simulink model "multiplex"  (R2020a)
settings: Solver=ode45  StartTime=0.0  StopTime=tiemposimu  RelTol=1e-3  EnableMultiTasking=on
values from neighbouring files (symbols this model uses):
  Atenuacion_canal = 22+20*log10(long2/lambda)-Gt-Gr    [Transmisor.m]
  Datos = length(codificacion)    [Transmisor.m]    (also in Transmisor2.m = length(codificacion3))
  frec = 2.5e6    (= 2500000)    [Transmisor.m]
  Frec1 = frec+0.25*Rb    (= 2531250)    [Transmisor.m]
  Frec2 = frec-0.25*Rb    (= 2468750)    [Transmisor.m]
  frec2 = 5e6    (= 5000000)    [Transmisor2.m]
  Frec3 = frec2+0.25*Rb    [Transmisor2.m]
  Frec4 = frec2-0.25*Rb    [Transmisor2.m]
  R1 = (kp*kv)/(wn^2*C)    (= 12.8228271575)    [Transmisor.m]
  R1C = 1/(R1*C)    (= 77985922.115)    [Transmisor.m]
  R2 = (2*zeta)/(wn*C)    (= 1028.57142857)    [Transmisor.m]
  Rb = 125e3    (= 125000)    [Transmisor.m]
  Retraso_canal = (long1/vp)+Ret_filtro    (= 1.30666666667e-05)    [Transmisor.m]
  Retraso_reloj = (0.1/Rb)    (= 8e-07)    [Transmisor.m]
libraries: commsynccomp2 x8, dspsigops x8, powerlib_meascontrol x6, dsparch4 x4, commnoisgen2 x3, simulink x2, dspsnks4 x2
settings Model: SimulationMode=accelerator  Creator=Maria Camila  LastModifiedBy=Usuario
settings DataIOCC: LimitDataPoints=on  SaveFormat=Array  ReturnWorkspaceOutputs=off
settings OptimizationCC: EfficientMapNaN2IntZero=off  LifeSpan=inf
settings DebuggingCC: UnderspecifiedInitializationDetection=Classic  MergeDetectMultiDrivingBlocksExec=none  SolverPrmCheckMsg=warning  SFUnexpectedBacktrackingDiag=warning  SFNoUnconditionalDefaultTransitionDiag=warning  SFExecutionAtInitializationDiag=none  ArithmeticOperatorsInVariantConditions=warning
settings HardwareCC: ProdBitPerPointer=32  ProdBitPerSizeT=32  ProdBitPerPtrDiffT=32  ProdLargestAtomicFloat=None  ProdIntDivRoundTo=Undefined  ProdEndianess=Unspecified  ProdWordSize=32  ProdHWDeviceType=32-bit Generic  TargetBitPerPointer=64  TargetBitPerSizeT=64  TargetBitPerPtrDiffT=64  TargetLongLongMode=on  TargetIntDivRoundTo=Zero  TargetEndianess=LittleEndian  TargetWordSize=64  TargetHWDeviceType=MATLAB Host  ProdEqTarget=off
settings ModelReferenceCC: PropagateSignalLabelsOutOfModel=off
settings SFSimCC: SimUseLocalCustomCode=off  CustomCodeUndefinedFunction=UseInterfaceOnly
settings RTWCC: RTWUseLocalCustomCode=off
settings CodeAppCC: MaxIdLength=128  StateflowObjectComments=on
settings GRTTargetCC: TargetLangStandard=C89/C90 (ANSI)  CombineOutputUpdateFcns=off  GRTInterface=on
settings ConfigComp: CovMetricSettings=dw  CovHtmlReporting=on  CovSaveCumulativeToWorkspaceVar=on  CovSaveSingleToWorkspaceVar=on  CovExternalEMLEnable=off
settings SimscapeCC: SimscapeNormalizeSystem=off
settings ConfigurationSet: Description=SimMechanics 2G

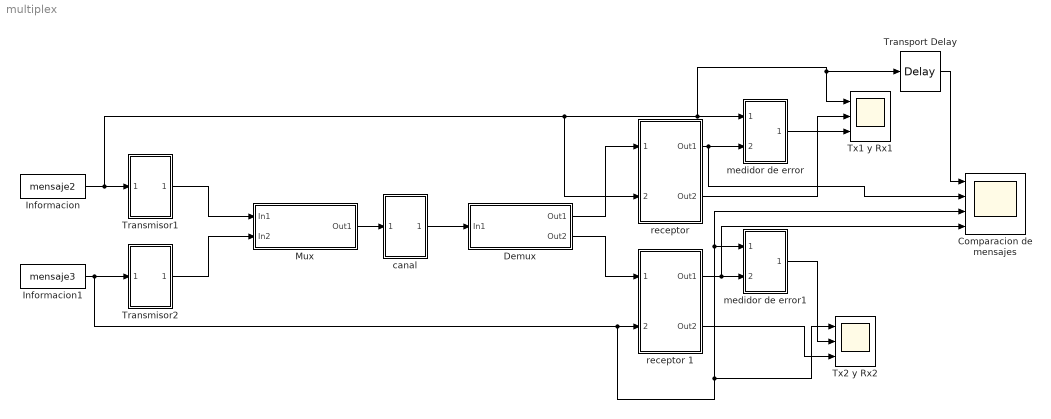
== system multiplex ==
  Comparacion de mensajes : Scope  NumInputPorts=4
  Demux : Subsystem
  Informacion : FromWorkspace  VariableName=mensaje2  SampleTime=1/Rb  Interpolate=off  OutputAfterFinalValue=Setting to zero
  Informacion1 : FromWorkspace  VariableName=mensaje3  SampleTime=1/Rb  Interpolate=off  OutputAfterFinalValue=Setting to zero
  Mux : Subsystem
  Transmisor1 : Subsystem
  Transmisor2 : Subsystem
  Transport Delay : TransportDelay  DelayTime=27.774e-6
  Tx1 y Rx1 : Scope  NumInputPorts=3
  Tx2 y Rx2 : Scope  NumInputPorts=3
  "canal " : Subsystem
  medidor de error : Subsystem
  medidor de error1 : Subsystem
  "receptor " : Subsystem
  receptor 1 : Subsystem
  wires:
  Mux/1(Out1) -> "canal "/1(In1)
  "canal "/1(Out1) -> Demux/1(In1)
  Transmisor2/1(Out1) -> Mux/2(In2)
  Transmisor1/1(Out1) -> Mux/1(In1)
  "receptor "/2(Out2) -> Tx1 y Rx1/2
  Informacion/1 -> Transmisor1/1(In1), "receptor "/2(Entada 2), Transport Delay/1, Tx1 y Rx1/1, medidor de error/1(In6)
  "receptor "/1(Out1) -> Comparacion de mensajes/2, medidor de error/2(In7)
  receptor 1/1(Out1) -> Comparacion de mensajes/4, medidor de error1/2(In7)
  medidor de error/1(Out1) -> Tx1 y Rx1/3
  receptor 1/2(Out2) -> Tx2 y Rx2/3
  medidor de error1/1(Out1) -> Tx2 y Rx2/2
  Informacion1/1 -> Comparacion de mensajes/3, medidor de error1/1(In6), Tx2 y Rx2/1, receptor 1/2(Entada 2), Transmisor2/1(In1)
  Demux/1(Out1) -> "receptor "/1(Entrada)
  Demux/2(Out2) -> receptor 1/1(Entrada)
  Transport Delay/1 -> Comparacion de mensajes/1

== system multiplex/Demux ==
  In1 : Inport
  Analog Filter Design : dsparch4/Analog Filter Design  method=Butterworth  filttype=Bandpass  N=5  Wlo=2*pi*(Frec2-Rb)  Whi=2*pi*(Frec1+Rb)  Rp=2  Rs=40
  Analog Filter Design2 : dsparch4/Analog Filter Design  method=Butterworth  filttype=Bandpass  N=5  Wlo=2*pi*(Frec4-Rb)  Whi=2*pi*(Frec3+Rb)  Rp=2  Rs=40
  Out1 : Outport
  Out2 : Outport  Port=2
  wires:
  In1/1 -> Analog Filter Design/1, Analog Filter Design2/1
  Analog Filter Design/1 -> Out1/1
  Analog Filter Design2/1 -> Out2/1

== system multiplex/Mux ==
  In1 : Inport
  In2 : Inport  Port=2
  Add : Sum
  Product : Product
  Product1 : Product
  Sine Wave : Sin  Frequency=2*pi*frec  SampleTime=0
  Sine Wave1 : Sin  Frequency=2*pi*frec2  SampleTime=0
  Out1 : Outport
  wires:
  Sine Wave/1 -> Product/2
  Sine Wave1/1 -> Product1/2
  Add/1 -> Out1/1
  Product1/1 -> Product1/1
  In2/1 -> Add/2
  In1/1 -> Add/1
  Product/1 -> Product/1

== system multiplex/Transmisor1 ==
  In1 : Inport
  Continuous-Time VCO : commsynccomp2/Continuous-Time VCO  Ac=1  Fc=Frec2  Kc=Rb/2  Ph=0
      settings: SourceProductBaseCode=CM
  Transport Delay : TransportDelay  DelayTime=0
  Out1 : Outport
  wires:
  In1/1 -> Transport Delay/1
  Continuous-Time VCO/1 -> Out1/1
  Transport Delay/1 -> Continuous-Time VCO/1

== system multiplex/Transmisor2 ==
  In1 : Inport
  Continuous-Time VCO : commsynccomp2/Continuous-Time VCO  Ac=1  Fc=Frec4  Kc=Rb/2  Ph=0
      settings: SourceProductBaseCode=CM
  Transport Delay : TransportDelay  DelayTime=0
  Out1 : Outport
  wires:
  In1/1 -> Transport Delay/1
  Continuous-Time VCO/1 -> Out1/1
  Transport Delay/1 -> Continuous-Time VCO/1

== system multiplex/canal  ==
  In1 : Inport
  Add : Sum
  Gain : Gain  Gain=1/Atenuacion_canal
  Gaussian Noise Generator : commnoisgen2/Gaussian Noise Generator  m=0  d=0  s=41  Ts=1e-9  frameBased=off  sampPerFrame=1  orient=off  outDataType=double
      settings: SourceProductBaseCode=CM
  Transport Delay : TransportDelay  DelayTime=Retraso_canal
  Out1 : Outport
  wires:
  In1/1 -> Gain/1
  Add/1 -> Out1/1
  Gain/1 -> Transport Delay/1
  Transport Delay/1 -> Add/1
  Gaussian Noise Generator/1 -> Add/2

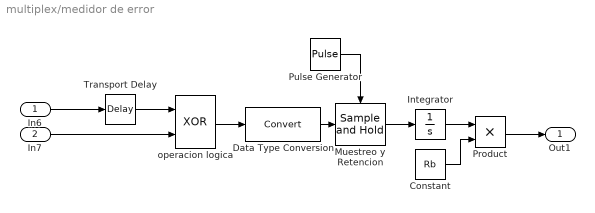
== system multiplex/medidor de error ==
  In6 : Inport
  In7 : Inport  Port=2
  Constant : Constant  Value=Rb
  Data Type Conversion : DataTypeConversion
  Integrator : Integrator
  "Muestreo y Retencion " : dspsigops/Sample and Hold  trig=Rising edge  initCond=0  latchinput=off
  Product : Product
  Pulse Generator : DiscretePulseGenerator  PulseType=Time based  Period=1/Rb  PhaseDelay=Retraso_reloj
  Transport Delay : TransportDelay  DelayTime=27.774e-6
  operacion logica : Logic  Operator=XOR  AllPortsSameDT=off  OutDataTypeStr=boolean
  Out1 : Outport
  wires:
  Product/1 -> Out1/1
  In6/1 -> Transport Delay/1
  operacion logica/1 -> Data Type Conversion/1
  Data Type Conversion/1 -> "Muestreo y Retencion "/1
  Constant/1 -> Product/2
  "Muestreo y Retencion "/1 -> Integrator/1
  Integrator/1 -> Product/1
  Pulse Generator/1 -> "Muestreo y Retencion "/Trigger
  In7/1 -> operacion logica/2
  Transport Delay/1 -> operacion logica/1

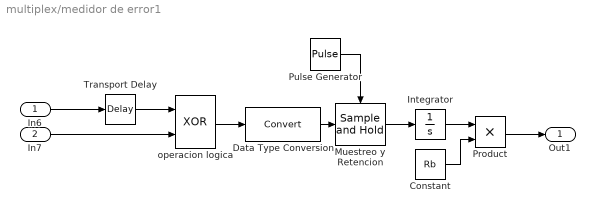
== system multiplex/medidor de error1 ==
  In6 : Inport
  In7 : Inport  Port=2
  Constant : Constant  Value=Rb
  Data Type Conversion : DataTypeConversion
  Integrator : Integrator
  "Muestreo y Retencion " : dspsigops/Sample and Hold  trig=Rising edge  initCond=0  latchinput=off
  Product : Product
  Pulse Generator : DiscretePulseGenerator  PulseType=Time based  Period=1/Rb  PhaseDelay=Retraso_reloj
  Transport Delay : TransportDelay  DelayTime=0.084e-4
  operacion logica : Logic  Operator=XOR  AllPortsSameDT=off  OutDataTypeStr=boolean
  Out1 : Outport
  wires:
  Product/1 -> Out1/1
  In6/1 -> Transport Delay/1
  operacion logica/1 -> Data Type Conversion/1
  Data Type Conversion/1 -> "Muestreo y Retencion "/1
  Constant/1 -> Product/2
  "Muestreo y Retencion "/1 -> Integrator/1
  Integrator/1 -> Product/1
  Pulse Generator/1 -> "Muestreo y Retencion "/Trigger
  In7/1 -> operacion logica/2
  Transport Delay/1 -> operacion logica/1

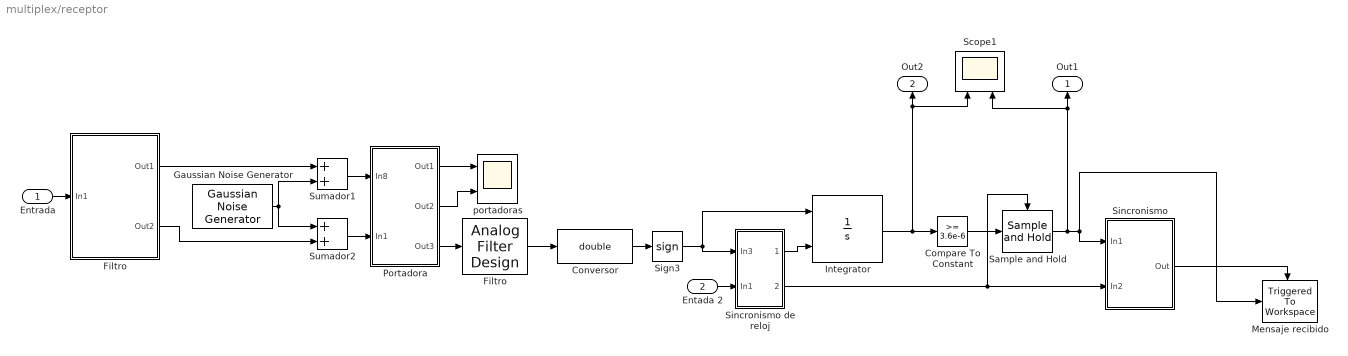
== system multiplex/receptor  ==
  Entrada : Inport
  Entada 2 : Inport  Port=2
  Compare To Constant : simulink/Logic and Bit Operations/Compare To Constant  relop=>=  const=3.6e-6  OutDataTypeStr=boolean
  Conversor : DataTypeConversion  OutDataTypeStr=double
  Filtro : dsparch4/Analog Filter Design  method=Butterworth  filttype=Lowpass  N=6  Wlo=2*pi*Rb  Whi=2*pi*(Frec1+Rb)  Rp=2  Rs=40
  "Filtro " : Subsystem
  Gaussian Noise Generator : commnoisgen2/Gaussian Noise Generator  m=0  d=Pot_ruido  s=41  Ts=1e-9  frameBased=off  sampPerFrame=1  orient=off  outDataType=double
      settings: SourceProductBaseCode=CM
  Integrator : Integrator  ExternalReset=either
  Mensaje recibido : dspsnks4/Triggered To Workspace  TriggerType=Either edge  VariableName=mensajerx2  Buffer=1000  Save2DMode=2-D array (concatenate along first dimension)
      settings: SourceProductBaseCode=DS  FixptAsFi=off
  "Portadora " : Subsystem
  Sample and Hold : dspsigops/Sample and Hold  trig=Either edge  initCond=0  latchinput=off
  Scope1 : Scope  NumInputPorts=2
  Sign3 : Signum
  "Sincronismo " : Subsystem
  Sincronismo de reloj : Subsystem
  Sumador1 : Sum
  Sumador2 : Sum
  portadoras : Scope  NumInputPorts=2
  Out1 : Outport
  Out2 : Outport  Port=2
  wires:
  Entrada/1 -> "Filtro "/1(In1)
  Sumador2/1 -> "Portadora "/2(In1)
  "Filtro "/1(Out1) -> Sumador1/1
  "Filtro "/2(Out2) -> Sumador2/2
  Gaussian Noise Generator/1 -> Sumador1/2, Sumador2/1
  Sumador1/1 -> "Portadora "/1(In8)
  "Portadora "/3(Out3) -> Filtro/1
  Sign3/1 -> Sincronismo de reloj/1(In3), Integrator/1
  Conversor/1 -> Sign3/1
  Integrator/1 -> Scope1/1, Out2/1, Compare To Constant/1
  Compare To Constant/1 -> Sample and Hold/1
  Sincronismo de reloj/2(Out2) -> Sample and Hold/Trigger, "Sincronismo "/2(In2)
  Sample and Hold/1 -> Scope1/2, Out1/1, "Sincronismo "/1(In1), Mensaje recibido/1
  Entada 2/1 -> Sincronismo de reloj/2(In1)
  Sincronismo de reloj/1(Out1) -> Integrator/2
  Filtro/1 -> Conversor/1
  "Sincronismo "/1("Out ") -> Mensaje recibido/Trigger
  "Portadora "/2(Out2) -> portadoras/2
  "Portadora "/1(Out1) -> portadoras/1

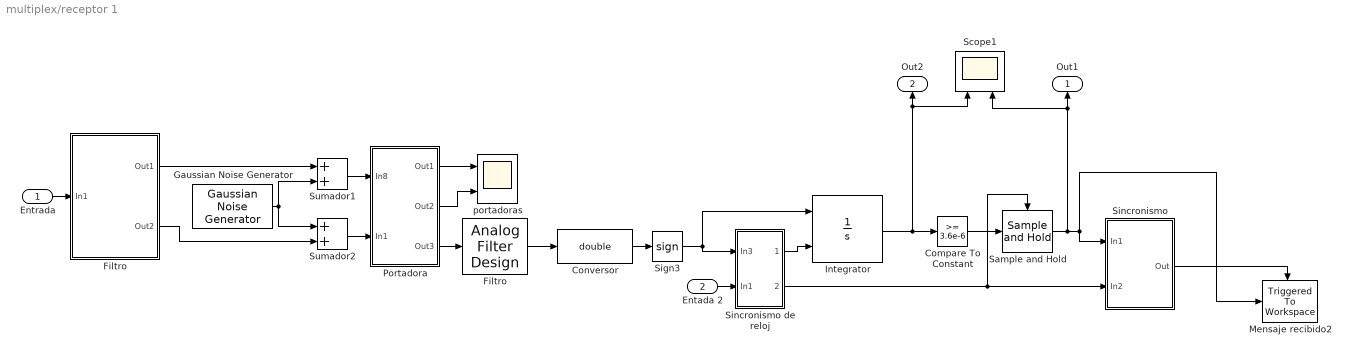
== system multiplex/receptor 1 ==
  Entrada : Inport
  Entada 2 : Inport  Port=2
  Compare To Constant : simulink/Logic and Bit Operations/Compare To Constant  relop=>=  const=3.6e-6  OutDataTypeStr=boolean
  Conversor : DataTypeConversion  OutDataTypeStr=double
  Filtro : dsparch4/Analog Filter Design  method=Butterworth  filttype=Lowpass  N=6  Wlo=2*pi*Rb  Whi=2*pi*(Frec1+Rb)  Rp=2  Rs=40
  "Filtro " : Subsystem
  Gaussian Noise Generator : commnoisgen2/Gaussian Noise Generator  m=0  d=Pot_ruido  s=41  Ts=1e-9  frameBased=off  sampPerFrame=1  orient=off  outDataType=double
      settings: SourceProductBaseCode=CM
  Integrator : Integrator  ExternalReset=either
  Mensaje recibido2 : dspsnks4/Triggered To Workspace  TriggerType=Either edge  VariableName=mensajerx3  Buffer=1000  Save2DMode=2-D array (concatenate along first dimension)
      settings: SourceProductBaseCode=DS  FixptAsFi=off
  "Portadora " : Subsystem
  Sample and Hold : dspsigops/Sample and Hold  trig=Either edge  initCond=0  latchinput=off
  Scope1 : Scope  NumInputPorts=2
  Sign3 : Signum
  "Sincronismo " : Subsystem
  Sincronismo de reloj : Subsystem
  Sumador1 : Sum
  Sumador2 : Sum
  portadoras : Scope  NumInputPorts=2
  Out1 : Outport
  Out2 : Outport  Port=2
  wires:
  Entrada/1 -> "Filtro "/1(In1)
  Sumador2/1 -> "Portadora "/2(In1)
  "Filtro "/1(Out1) -> Sumador1/1
  "Filtro "/2(Out2) -> Sumador2/2
  Gaussian Noise Generator/1 -> Sumador1/2, Sumador2/1
  Sumador1/1 -> "Portadora "/1(In8)
  "Portadora "/3(Out3) -> Filtro/1
  Sign3/1 -> Sincronismo de reloj/1(In3), Integrator/1
  Conversor/1 -> Sign3/1
  Integrator/1 -> Scope1/1, Out2/1, Compare To Constant/1
  Compare To Constant/1 -> Sample and Hold/1
  Sincronismo de reloj/2(Out2) -> Sample and Hold/Trigger, "Sincronismo "/2(In2)
  Sample and Hold/1 -> Scope1/2, Out1/1, "Sincronismo "/1(In1), Mensaje recibido2/1
  Entada 2/1 -> Sincronismo de reloj/2(In1)
  Sincronismo de reloj/1(Out1) -> Integrator/2
  Filtro/1 -> Conversor/1
  "Sincronismo "/1("Out ") -> Mensaje recibido2/Trigger
  "Portadora "/2(Out2) -> portadoras/2
  "Portadora "/1(Out1) -> portadoras/1

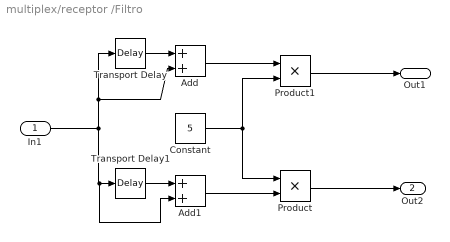
== system multiplex/receptor /Filtro  ==
  In1 : Inport
  Add : Sum
  Add1 : Sum
  Constant : Constant  Value=5
  Product : Product
  Product1 : Product
  Transport Delay : TransportDelay  DelayTime=0.5/Frec2
  Transport Delay1 : TransportDelay  DelayTime=0.5/Frec1
  Out1 : Outport
  Out2 : Outport  Port=2
  wires:
  Add/1 -> Product1/1
  Add1/1 -> Product/2
  Constant/1 -> Product/1, Product1/2
  Transport Delay1/1 -> Add1/1
  Transport Delay/1 -> Add/1
  In1/1 -> Add1/2, Transport Delay1/1, Add/2, Transport Delay/1
  Product/1 -> Out2/1
  Product1/1 -> Out1/1

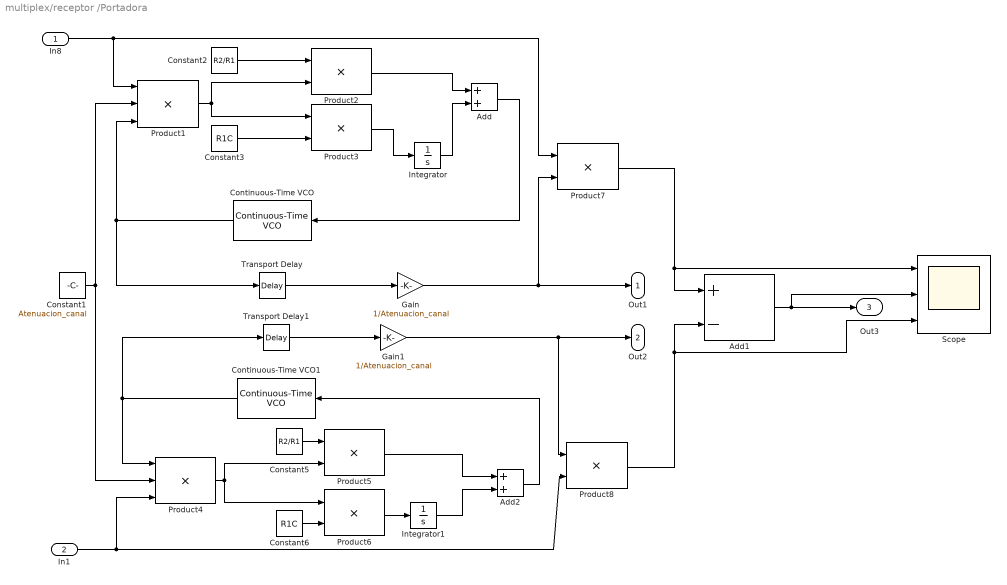
== system multiplex/receptor /Portadora  ==
  In8 : Inport
  In1 : Inport  Port=2
  Add : Sum
  Add1 : Sum  Inputs=+-
  Add2 : Sum
  Constant1 : Constant  Value=Atenuacion_canal
  Constant2 : Constant  Value=R2/R1
  Constant3 : Constant  Value=R1C
  Constant5 : Constant  Value=R2/R1
  Constant6 : Constant  Value=R1C
  Continuous-Time VCO : commsynccomp2/Continuous-Time VCO  Ac=1  Fc=Frec1  Kc=kv  Ph=0
      settings: SourceProductBaseCode=CM
  Continuous-Time VCO1 : commsynccomp2/Continuous-Time VCO  Ac=1  Fc=Frec2  Kc=kv  Ph=0
      settings: SourceProductBaseCode=CM
  Gain : Gain  Gain=1/Atenuacion_canal
  Gain1 : Gain  Gain=1/Atenuacion_canal
  Integrator : Integrator
  Integrator1 : Integrator
  Product1 : Product  Inputs=3
  Product{2..3,5..8} (6 alike) : Product
  Product4 : Product  Inputs=3
  Scope : Scope  NumInputPorts=3
  Transport Delay : TransportDelay  DelayTime=0.25/Frec1
  Transport Delay1 : TransportDelay  DelayTime=0.25/Frec2
  Out1 : Outport
  Out2 : Outport  Port=2
  Out3 : Outport  Port=3
  wires:
  Constant2/1 -> Product2/1
  Product1/1 -> Product3/1, Product2/2
  Integrator/1 -> Add/2
  Continuous-Time VCO/1 -> Transport Delay/1, Product1/3
  Transport Delay/1 -> Gain/1
  Product3/1 -> Integrator/1
  Product2/1 -> Add/1
  Constant3/1 -> Product3/2
  Integrator1/1 -> Add2/2
  Constant5/1 -> Product5/1
  Product4/1 -> Product6/1, Product5/2
  Continuous-Time VCO1/1 -> Product4/1, Transport Delay1/1
  Add2/1 -> Continuous-Time VCO1/1
  Transport Delay1/1 -> Gain1/1
  Product6/1 -> Integrator1/1
  Product5/1 -> Add2/1
  Constant6/1 -> Product6/2
  Add/1 -> Continuous-Time VCO/1
  In8/1 -> Product1/1, Product7/1
  Constant1/1 -> Product4/2, Product1/2
  In1/1 -> Product8/2, Product4/3
  Gain/1 -> Out1/1, Product7/2
  Gain1/1 -> Product8/1, Out2/1
  Add1/1 -> Out3/1, Scope/2
  Product7/1 -> Add1/1, Scope/1
  Product8/1 -> Scope/3, Add1/2

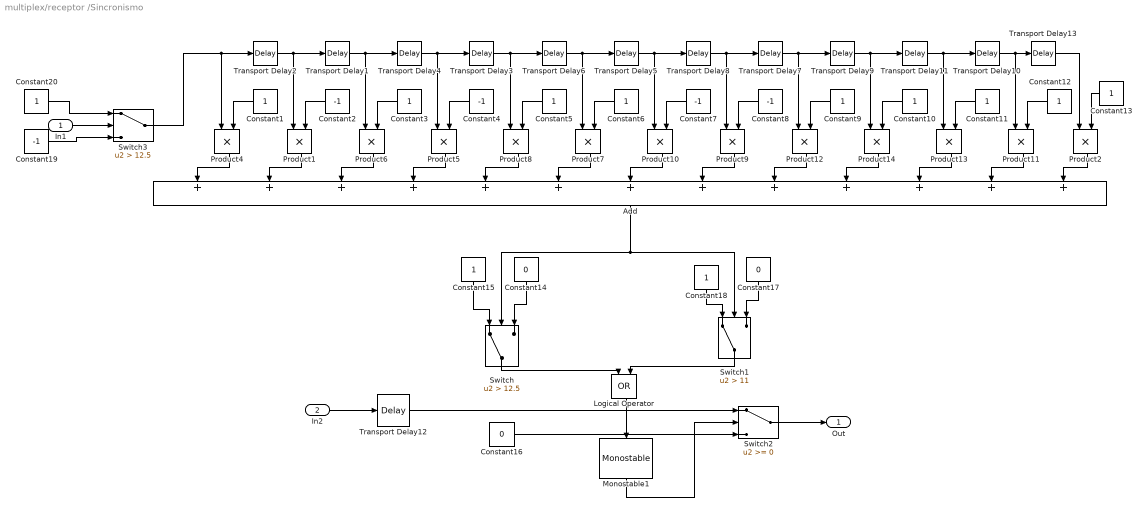
== system multiplex/receptor /Sincronismo  ==
  In1 : Inport
  In2 : Inport  Port=2
  Add : Sum  Inputs=+++++++++++++
  Constant{1,3,5..6,9..13,15,18,20} (12 alike) : Constant
  Constant14 : Constant  Value=0
  Constant16 : Constant  Value=0
  Constant17 : Constant  Value=0
  Constant{2,4,7..8,19} (5 alike) : Constant  Value=-1
  Logical Operator : Logic  Operator=OR  AllPortsSameDT=off  OutDataTypeStr=boolean
  Monostable1 : powerlib_meascontrol/Logic/Monostable  EdgeDetect=Rising  PulseDuration=(Datos+0)/Rb  ic=0  Ts=0
      settings: SourceProductBaseCode=PS
  Product{1..2,4..14} (13 alike) : Product
  Switch : Switch  Criteria=u2 > Threshold  Threshold=12.5
  Switch1 : Switch  Criteria=u2 > Threshold  Threshold=11
  Switch2 : Switch
  Switch3 : Switch  Criteria=u2 > Threshold  Threshold=12.5
  Transport Delay{1..11,13} (12 alike) : TransportDelay  DelayTime=1/Rb
  Transport Delay12 : TransportDelay  DelayTime=0
  "Out " : Outport
  wires:
  Transport Delay10/1 -> Transport Delay13/1, Product11/1
  Transport Delay1/1 -> Product6/1, Transport Delay4/1
  Constant2/1 -> Product1/2
  Product1/1 -> Add/2
  Transport Delay5/1 -> Product10/1, Transport Delay8/1
  Transport Delay11/1 -> Product13/1, Transport Delay10/1
  Product11/1 -> Add/12
  Constant11/1 -> Product13/2
  Product13/1 -> Add/11
  Transport Delay7/1 -> Product12/1, Transport Delay9/1
  Constant10/1 -> Product14/2
  Constant9/1 -> Product12/2
  Product14/1 -> Add/10
  Product12/1 -> Add/9
  Product4/1 -> Add/1
  Transport Delay3/1 -> Product8/1, Transport Delay6/1
  Product8/1 -> Add/5
  Product7/1 -> Add/6
  Product9/1 -> Add/8
  Constant5/1 -> Product8/2
  Constant6/1 -> Product7/2
  Transport Delay8/1 -> Product9/1, Transport Delay7/1
  Product10/1 -> Add/7
  Transport Delay6/1 -> Product7/1, Transport Delay5/1
  Constant7/1 -> Product10/2
  Constant8/1 -> Product9/2
  Constant1/1 -> Product4/2
  Transport Delay2/1 -> Product1/1, Transport Delay1/1
  Product5/1 -> Add/4
  Transport Delay4/1 -> Product5/1, Transport Delay3/1
  Constant3/1 -> Product6/2
  Constant4/1 -> Product5/2
  Product6/1 -> Add/3
  Constant15/1 -> Switch/1
  Transport Delay9/1 -> Product14/1, Transport Delay11/1
  Constant14/1 -> Switch/3
  Constant18/1 -> Switch1/1
  Constant17/1 -> Switch1/3
  Switch/1 -> Logical Operator/1
  Switch1/1 -> Logical Operator/2
  Logical Operator/1 -> Monostable1/1
  Monostable1/1 -> Switch2/2
  Constant16/1 -> Switch2/3
  In2/1 -> Transport Delay12/1
  Transport Delay12/1 -> Switch2/1
  Switch2/1 -> "Out "/1
  Add/1 -> Switch1/2, Switch/2
  Constant20/1 -> Switch3/1
  Constant19/1 -> Switch3/3
  In1/1 -> Switch3/2
  Switch3/1 -> Product4/1, Transport Delay2/1
  Constant12/1 -> Product11/2
  Product2/1 -> Add/13
  Constant13/1 -> Product2/2
  Transport Delay13/1 -> Product2/1

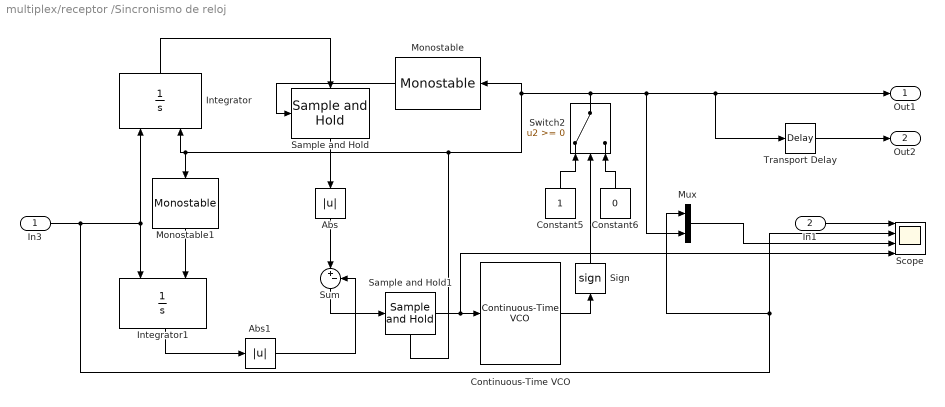
== system multiplex/receptor /Sincronismo de reloj ==
  In3 : Inport
  In1 : Inport  Port=2
  Abs : Abs
  Abs1 : Abs
  Constant5 : Constant
  Constant6 : Constant  Value=0
  Continuous-Time VCO : commsynccomp2/Continuous-Time VCO  Ac=1  Fc=Rb/2  Kc=kv2  Ph=0
      settings: SourceProductBaseCode=CM
  Integrator : Integrator  ExternalReset=either
  Integrator1 : Integrator  ExternalReset=falling
  Monostable : powerlib_meascontrol/Logic/Monostable  EdgeDetect=Either  PulseDuration=0.9/Rb  ic=0  Ts=0
      settings: SourceProductBaseCode=PS
  Monostable1 : powerlib_meascontrol/Logic/Monostable  EdgeDetect=Either  PulseDuration=0.1/Rb  ic=0  Ts=0
      settings: SourceProductBaseCode=PS
  Mux : Mux  Inputs=2
  Sample and Hold : dspsigops/Sample and Hold  trig=Falling edge  initCond=0  latchinput=off
  Sample and Hold1 : dspsigops/Sample and Hold  trig=Either edge  initCond=0  latchinput=off
  Scope : Scope  NumInputPorts=4
  Sign : Signum
  Sum : Sum  Inputs=|+-
  Switch2 : Switch
  Transport Delay : TransportDelay  DelayTime=(0.95/Rb)
  Out1 : Outport
  Out2 : Outport  Port=2
  wires:
  Monostable1/1 -> Integrator1/2
  Integrator1/1 -> Abs1/1
  Mux/1 -> Scope/3
  Continuous-Time VCO/1 -> Sign/1
  In3/1 -> Mux/1, Scope/2, Integrator/1, Integrator1/1
  Integrator/1 -> Sample and Hold/1
  Sample and Hold/1 -> Abs/1
  Sample and Hold1/1 -> Scope/4, Continuous-Time VCO/1
  Monostable/1 -> Sample and Hold/Trigger
  In1/1 -> Scope/1
  Constant5/1 -> Switch2/1
  Constant6/1 -> Switch2/3
  Sign/1 -> Switch2/2
  Switch2/1 -> Transport Delay/1, Out1/1, Mux/2, Monostable1/1, Integrator/2, Sample and Hold1/Trigger, Monostable/1
  Abs/1 -> Sum/1
  Sum/1 -> Sample and Hold1/1
  Abs1/1 -> Sum/2
  Transport Delay/1 -> Out2/1

== system multiplex/receptor 1/Filtro  ==
  In1 : Inport
  Add : Sum
  Add1 : Sum
  Constant : Constant  Value=5
  Product : Product
  Product1 : Product
  Transport Delay : TransportDelay  DelayTime=0.5/Frec4
  Transport Delay1 : TransportDelay  DelayTime=0.5/Frec3
  Out1 : Outport
  Out2 : Outport  Port=2
  wires:
  Add/1 -> Product1/1
  Add1/1 -> Product/2
  Constant/1 -> Product/1, Product1/2
  Transport Delay1/1 -> Add1/1
  Transport Delay/1 -> Add/1
  In1/1 -> Add1/2, Transport Delay1/1, Add/2, Transport Delay/1
  Product/1 -> Out2/1
  Product1/1 -> Out1/1

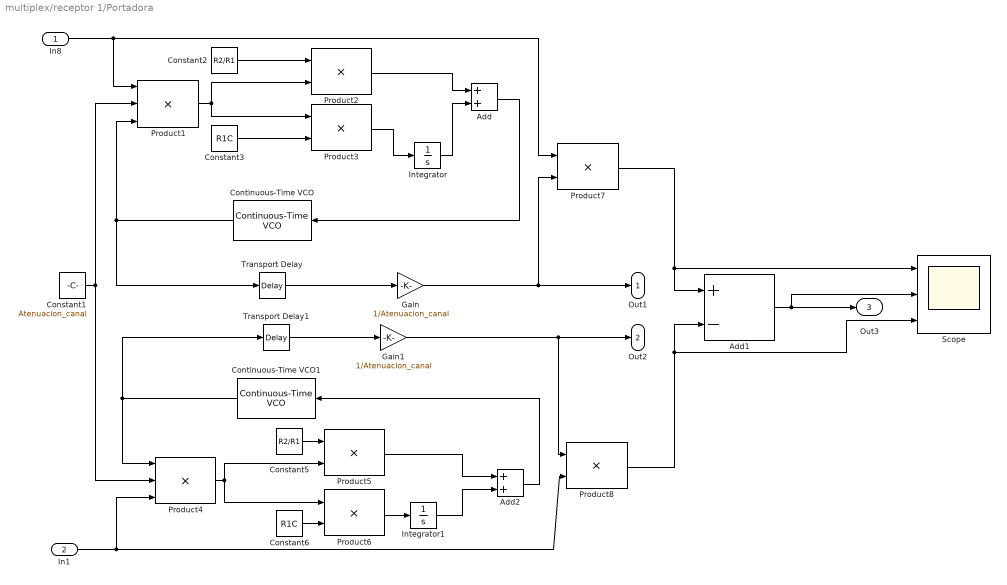
== system multiplex/receptor 1/Portadora  ==
  In8 : Inport
  In1 : Inport  Port=2
  Add : Sum
  Add1 : Sum  Inputs=+-
  Add2 : Sum
  Constant1 : Constant  Value=Atenuacion_canal
  Constant2 : Constant  Value=R2/R1
  Constant3 : Constant  Value=R1C
  Constant5 : Constant  Value=R2/R1
  Constant6 : Constant  Value=R1C
  Continuous-Time VCO : commsynccomp2/Continuous-Time VCO  Ac=1  Fc=Frec3  Kc=kv  Ph=0
      settings: SourceProductBaseCode=CM
  Continuous-Time VCO1 : commsynccomp2/Continuous-Time VCO  Ac=1  Fc=Frec4  Kc=kv  Ph=0
      settings: SourceProductBaseCode=CM
  Gain : Gain  Gain=1/Atenuacion_canal
  Gain1 : Gain  Gain=1/Atenuacion_canal
  Integrator : Integrator
  Integrator1 : Integrator
  Product1 : Product  Inputs=3
  Product{2..3,5..8} (6 alike) : Product
  Product4 : Product  Inputs=3
  Scope : Scope  NumInputPorts=3
  Transport Delay : TransportDelay  DelayTime=0.25/Frec3
  Transport Delay1 : TransportDelay  DelayTime=0.25/Frec4
  Out1 : Outport
  Out2 : Outport  Port=2
  Out3 : Outport  Port=3
  wires:
  Constant2/1 -> Product2/1
  Product1/1 -> Product3/1, Product2/2
  Integrator/1 -> Add/2
  Continuous-Time VCO/1 -> Transport Delay/1, Product1/3
  Transport Delay/1 -> Gain/1
  Product3/1 -> Integrator/1
  Product2/1 -> Add/1
  Constant3/1 -> Product3/2
  Integrator1/1 -> Add2/2
  Constant5/1 -> Product5/1
  Product4/1 -> Product6/1, Product5/2
  Continuous-Time VCO1/1 -> Product4/1, Transport Delay1/1
  Add2/1 -> Continuous-Time VCO1/1
  Transport Delay1/1 -> Gain1/1
  Product6/1 -> Integrator1/1
  Product5/1 -> Add2/1
  Constant6/1 -> Product6/2
  Add/1 -> Continuous-Time VCO/1
  In8/1 -> Product1/1, Product7/1
  Constant1/1 -> Product4/2, Product1/2
  In1/1 -> Product8/2, Product4/3
  Gain/1 -> Out1/1, Product7/2
  Gain1/1 -> Product8/1, Out2/1
  Add1/1 -> Out3/1, Scope/2
  Product7/1 -> Add1/1, Scope/1
  Product8/1 -> Scope/3, Add1/2

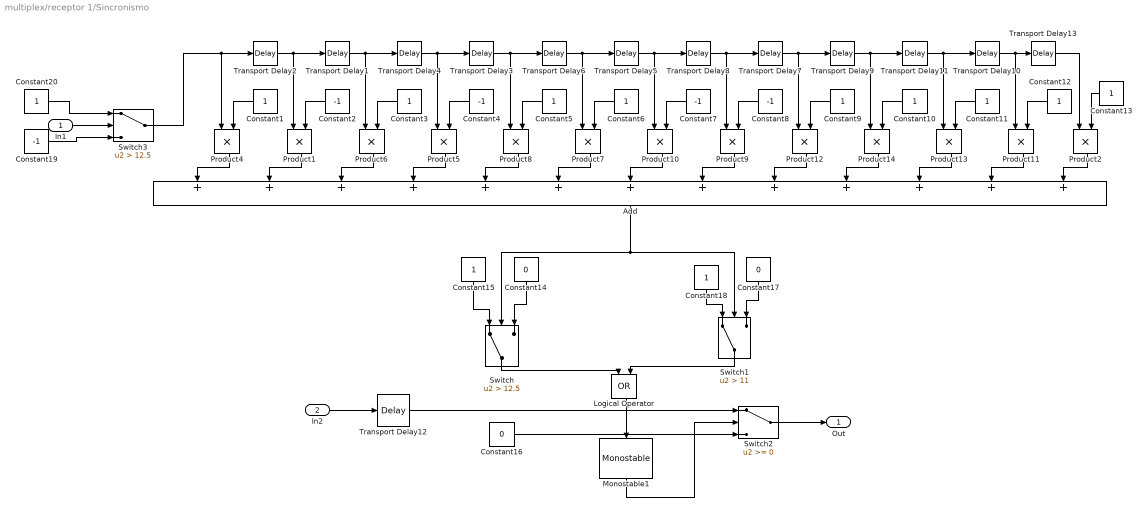
== system multiplex/receptor 1/Sincronismo  ==
  In1 : Inport
  In2 : Inport  Port=2
  Add : Sum  Inputs=+++++++++++++
  Constant{1,3,5..6,9..13,15,18,20} (12 alike) : Constant
  Constant14 : Constant  Value=0
  Constant16 : Constant  Value=0
  Constant17 : Constant  Value=0
  Constant{2,4,7..8,19} (5 alike) : Constant  Value=-1
  Logical Operator : Logic  Operator=OR  AllPortsSameDT=off  OutDataTypeStr=boolean
  Monostable1 : powerlib_meascontrol/Logic/Monostable  EdgeDetect=Rising  PulseDuration=(Datos+0)/Rb  ic=0  Ts=0
      settings: SourceProductBaseCode=PS
  Product{1..2,4..14} (13 alike) : Product
  Switch : Switch  Criteria=u2 > Threshold  Threshold=12.5
  Switch1 : Switch  Criteria=u2 > Threshold  Threshold=11
  Switch2 : Switch
  Switch3 : Switch  Criteria=u2 > Threshold  Threshold=12.5
  Transport Delay{1..11,13} (12 alike) : TransportDelay  DelayTime=1/Rb
  Transport Delay12 : TransportDelay  DelayTime=0
  "Out " : Outport
  wires:
  Transport Delay10/1 -> Transport Delay13/1, Product11/1
  Transport Delay1/1 -> Product6/1, Transport Delay4/1
  Constant2/1 -> Product1/2
  Product1/1 -> Add/2
  Transport Delay5/1 -> Product10/1, Transport Delay8/1
  Transport Delay11/1 -> Product13/1, Transport Delay10/1
  Product11/1 -> Add/12
  Constant11/1 -> Product13/2
  Product13/1 -> Add/11
  Transport Delay7/1 -> Product12/1, Transport Delay9/1
  Constant10/1 -> Product14/2
  Constant9/1 -> Product12/2
  Product14/1 -> Add/10
  Product12/1 -> Add/9
  Product4/1 -> Add/1
  Transport Delay3/1 -> Product8/1, Transport Delay6/1
  Product8/1 -> Add/5
  Product7/1 -> Add/6
  Product9/1 -> Add/8
  Constant5/1 -> Product8/2
  Constant6/1 -> Product7/2
  Transport Delay8/1 -> Product9/1, Transport Delay7/1
  Product10/1 -> Add/7
  Transport Delay6/1 -> Product7/1, Transport Delay5/1
  Constant7/1 -> Product10/2
  Constant8/1 -> Product9/2
  Constant1/1 -> Product4/2
  Transport Delay2/1 -> Product1/1, Transport Delay1/1
  Product5/1 -> Add/4
  Transport Delay4/1 -> Product5/1, Transport Delay3/1
  Constant3/1 -> Product6/2
  Constant4/1 -> Product5/2
  Product6/1 -> Add/3
  Constant15/1 -> Switch/1
  Transport Delay9/1 -> Product14/1, Transport Delay11/1
  Constant14/1 -> Switch/3
  Constant18/1 -> Switch1/1
  Constant17/1 -> Switch1/3
  Switch/1 -> Logical Operator/1
  Switch1/1 -> Logical Operator/2
  Logical Operator/1 -> Monostable1/1
  Monostable1/1 -> Switch2/2
  Constant16/1 -> Switch2/3
  In2/1 -> Transport Delay12/1
  Transport Delay12/1 -> Switch2/1
  Switch2/1 -> "Out "/1
  Add/1 -> Switch1/2, Switch/2
  Constant20/1 -> Switch3/1
  Constant19/1 -> Switch3/3
  In1/1 -> Switch3/2
  Switch3/1 -> Product4/1, Transport Delay2/1
  Constant12/1 -> Product11/2
  Product2/1 -> Add/13
  Constant13/1 -> Product2/2
  Transport Delay13/1 -> Product2/1

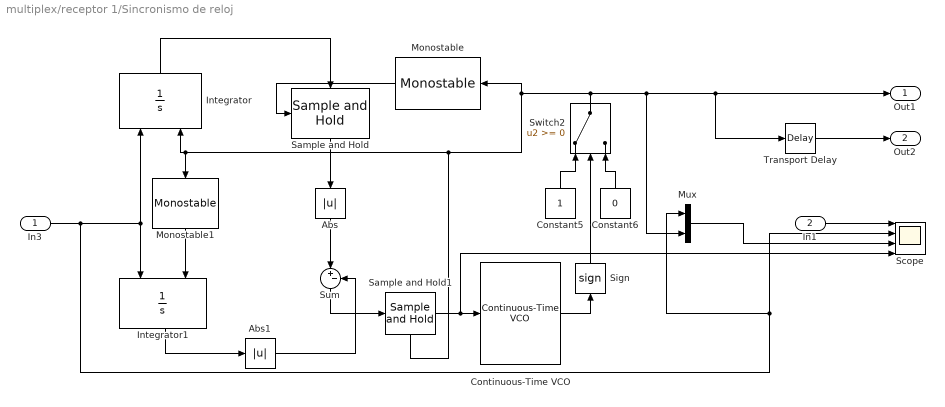
== system multiplex/receptor 1/Sincronismo de reloj ==
  In3 : Inport
  In1 : Inport  Port=2
  Abs : Abs
  Abs1 : Abs
  Constant5 : Constant
  Constant6 : Constant  Value=0
  Continuous-Time VCO : commsynccomp2/Continuous-Time VCO  Ac=1  Fc=Rb/2  Kc=kv2  Ph=0
      settings: SourceProductBaseCode=CM
  Integrator : Integrator  ExternalReset=either
  Integrator1 : Integrator  ExternalReset=falling
  Monostable : powerlib_meascontrol/Logic/Monostable  EdgeDetect=Either  PulseDuration=0.9/Rb  ic=0  Ts=0
      settings: SourceProductBaseCode=PS
  Monostable1 : powerlib_meascontrol/Logic/Monostable  EdgeDetect=Either  PulseDuration=0.1/Rb  ic=0  Ts=0
      settings: SourceProductBaseCode=PS
  Mux : Mux  Inputs=2
  Sample and Hold : dspsigops/Sample and Hold  trig=Falling edge  initCond=0  latchinput=off
  Sample and Hold1 : dspsigops/Sample and Hold  trig=Either edge  initCond=0  latchinput=off
  Scope : Scope  NumInputPorts=4
  Sign : Signum
  Sum : Sum  Inputs=|+-
  Switch2 : Switch
  Transport Delay : TransportDelay  DelayTime=(0.95/Rb)
  Out1 : Outport
  Out2 : Outport  Port=2
  wires:
  Monostable1/1 -> Integrator1/2
  Integrator1/1 -> Abs1/1
  Mux/1 -> Scope/3
  Continuous-Time VCO/1 -> Sign/1
  In3/1 -> Mux/1, Scope/2, Integrator/1, Integrator1/1
  Integrator/1 -> Sample and Hold/1
  Sample and Hold/1 -> Abs/1
  Sample and Hold1/1 -> Scope/4, Continuous-Time VCO/1
  Monostable/1 -> Sample and Hold/Trigger
  In1/1 -> Scope/1
  Constant5/1 -> Switch2/1
  Constant6/1 -> Switch2/3
  Sign/1 -> Switch2/2
  Switch2/1 -> Transport Delay/1, Out1/1, Mux/2, Monostable1/1, Integrator/2, Sample and Hold1/Trigger, Monostable/1
  Abs/1 -> Sum/1
  Sum/1 -> Sample and Hold1/1
  Abs1/1 -> Sum/2
  Transport Delay/1 -> Out2/1
